simulink model "IP_Nonlinear_model"  (R2022a)
settings: Solver=FixedStepAuto  StartTime=0.0  StopTime=inf  FixedStep=0.01  RelTol=1e-3
InitFcn:
  | M = 0.5;
  | m = 0.5;
  | l = 0.3;
  | I = 0.006;
  | mu = 0.1;
  | g = 9.81
undefined symbols (not defined in the file): denC, numC
libraries: vrlib x3
settings Model: Creator=jitendra  LastModifiedBy=vcichella
settings DataIOCC: ExternalInput=getinputstruct(op_trim1)  InitialState=getstatestruct(op_trim1)  ReturnWorkspaceOutputs=off
settings DebuggingCC: UnconnectedInputMsg=warning  UnconnectedOutputMsg=warning  UnconnectedLineMsg=warning  SFMachineParentedDataDiag=warning  ArithmeticOperatorsInVariantConditions=warning
settings SFSimCC: SimUseLocalCustomCode=off  CustomCodeUndefinedFunction=UseInterfaceOnly
settings RTWCC: RTWUseLocalCustomCode=off

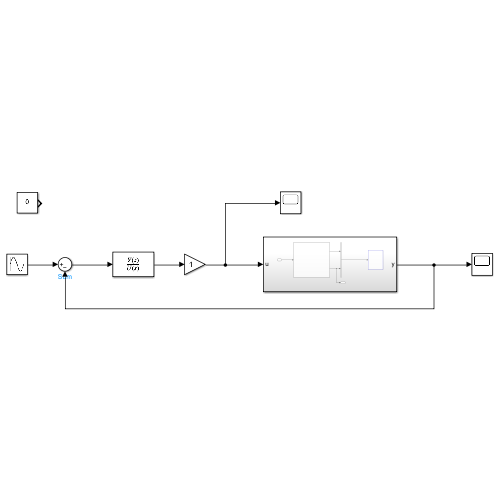
[thumbnail: Simulink's stored preview of the top-level diagram]
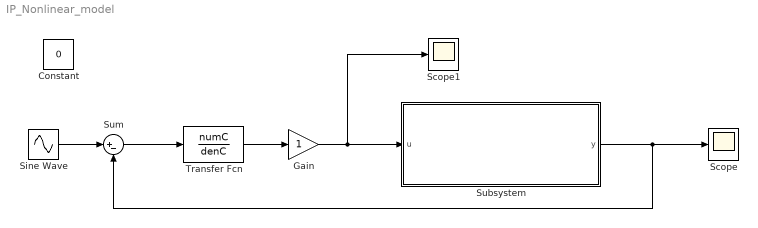
== system IP_Nonlinear_model ==
  Constant : Constant  Value=0
  Gain : Gain
  Scope : Scope
  Scope1 : Scope
  Sine Wave : Sin  Amplitude=0.1  Frequency=20  SampleTime=0
  Subsystem : Subsystem
  Sum : Sum  Inputs=|+-
  Transfer Fcn : TransferFcn  Numerator=numC  Denominator=denC
  wires:
  Sum/1 -> Transfer Fcn/1
  Subsystem/1(y) -> Scope/1, Sum/2
  Transfer Fcn/1 -> Gain/1
  Gain/1 -> Subsystem/1(u), Scope1/1
  Sine Wave/1 -> Sum/1

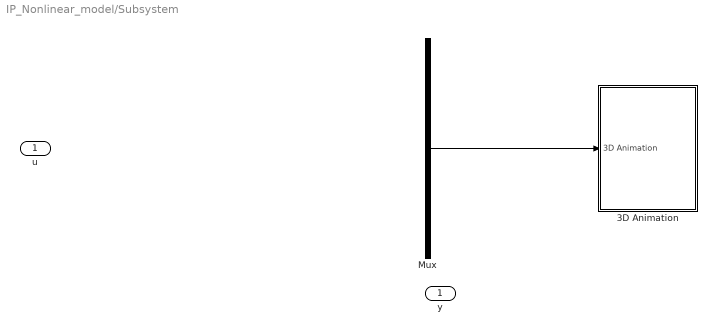
== system IP_Nonlinear_model/Subsystem ==
  u : Inport
  3D Animation : Subsystem
  Mux : Mux  Inputs=2
  y : Outport
  wires:
  Mux/1 -> 3D Animation/1(3D Animation)
  ? -> y/1, Mux/2  "theta"
  ? -> Mux/1  "X"

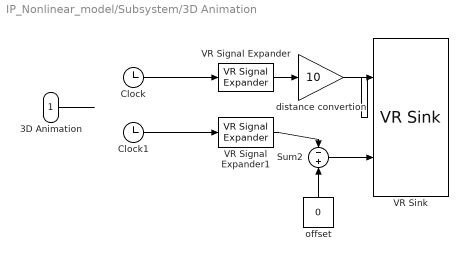
== system IP_Nonlinear_model/Subsystem/3D Animation ==
  3D Animation : Inport
  Clock : Clock
  Clock1 : Clock
  Sum2 : Sum  Inputs=-|+
  VR Signal Expander : vrlib/VR Signal Expander  outwidth=3  outidx=[1]
  VR Signal Expander1 : vrlib/VR Signal Expander  outwidth=4  outidx=[4]
  VR Sink : vrlib/VR Sink  InstantiateOnLoad=on  SampleTime=0.02  ViewEnable=on  RemoteChange=off  RemoteView=off  FieldsWritten=joint.rotation.4.1.1.double#rod.rotation.4.1.1.double  WorldFileName=InvertedPendulum.wrl  AutoView=on  VideoDimensions=[]  AllowVariableSize=off
  distance convertion : Gain  Gain=10
  offset : Constant  Value=0
  wires:
  VR Signal Expander/1 -> distance convertion/1
  3D Animation/1 -> ?
  offset/1 -> Sum2/2
  VR Signal Expander1/1 -> Sum2/1
  distance convertion/1 -> VR Sink/1
  Clock/1 -> VR Signal Expander/1
  Clock1/1 -> VR Signal Expander1/1
  Sum2/1 -> VR Sink/2
